simulink model "Golden_Model"  (R2025b)
settings: Solver=VariableStepAuto  StartTime=0.0  StopTime=20  RelTol=1e-3
undefined symbols (not defined in the file): b_mech, g, K_force, Kd_x_dummy, Ki_i_dummy, Kp_i_dummy, Kp_x_dummy, L, m, R_coil, R_eff
settings Model: Creator=nektariakaragiannis  LastModifiedBy=lucianbracy

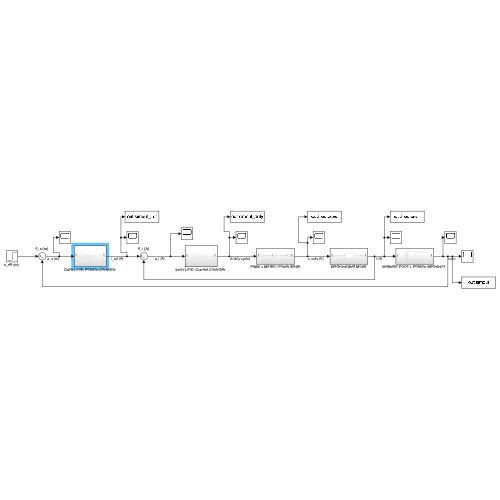
[thumbnail: Simulink's stored preview of the top-level diagram]
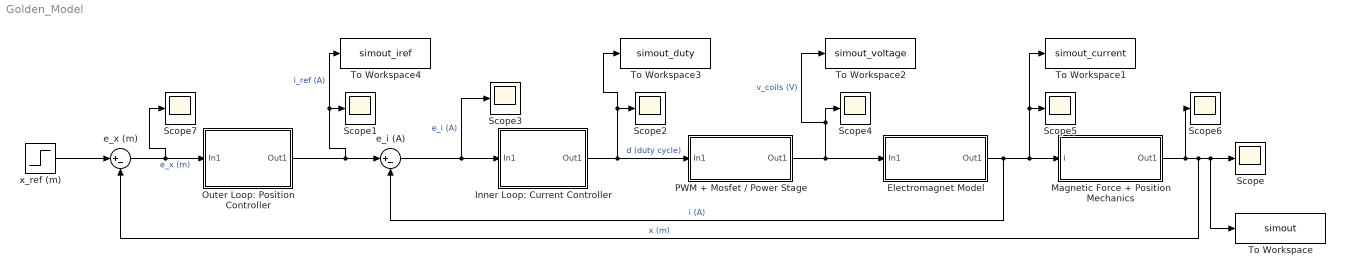
== system Golden_Model ==
  Electromagnet Model : Subsystem
  "Inner Loop: Current Controller " : Subsystem
  "Magnetic Force + Position Mechanics " : Subsystem
  Outer Loop: Position Controller : Subsystem
  PWM + Mosfet / Power Stage : Subsystem
  Scope{,1..7} (8 alike) : Scope
      Scope settings: ActiveDisplayYMinimum=-1  ActiveDisplayYMaximum=1
      Scope1 settings: ActiveDisplayYMinimum=-1  ActiveDisplayYMaximum=1  DataLoggingVariableName=ScopeData3
      Scope2 settings: ActiveDisplayYMinimum=-1  ActiveDisplayYMaximum=1  DataLoggingVariableName=ScopeData4
      Scope3 settings: ActiveDisplayYMinimum=-1  ActiveDisplayYMaximum=1  DataLoggingVariableName=ScopeData5
      Scope4 settings: ActiveDisplayYMinimum=-1  ActiveDisplayYMaximum=1  DataLoggingVariableName=ScopeData6
      Scope5 settings: ActiveDisplayYMinimum=-1  ActiveDisplayYMaximum=1  DataLoggingVariableName=ScopeData7
      Scope6 settings: ActiveDisplayYMinimum=-1  ActiveDisplayYMaximum=1  DataLoggingVariableName=ScopeData8
      Scope7 settings: ActiveDisplayYMinimum=-1  ActiveDisplayYMaximum=1  DataLoggingVariableName=ScopeData9
  To Workspace : ToWorkspace  VariableName=simout  SaveFormat=Timeseries  SampleTime=-1
  To Workspace1 : ToWorkspace  VariableName=simout_current  SaveFormat=Timeseries  SampleTime=-1
  To Workspace2 : ToWorkspace  VariableName=simout_voltage  SaveFormat=Timeseries  SampleTime=-1
  To Workspace3 : ToWorkspace  VariableName=simout_duty  SaveFormat=Timeseries  SampleTime=-1
  To Workspace4 : ToWorkspace  VariableName=simout_iref  SaveFormat=Timeseries  SampleTime=-1
  e_i (A) : Sum  Inputs=|+-
  e_x (m) : Sum  Inputs=|+-
  "x_ref (m) " : Step  After=0.0127  SampleTime=0
  wires:
  "x_ref (m) "/1 -> e_x (m)/1
  e_x (m)/1 -> Scope7/1, Outer Loop: Position Controller/1(In1)  "e_x (m)"
  Outer Loop: Position Controller/1(Out1) -> To Workspace4/1, Scope1/1, e_i (A)/1  "i_ref (A)"
  e_i (A)/1 -> Scope3/1, "Inner Loop: Current Controller "/1(In1)  "e_i (A)"
  "Inner Loop: Current Controller "/1(Out1) -> To Workspace3/1, Scope2/1, PWM + Mosfet / Power Stage/1(In1)  "d (duty cycle)"
  PWM + Mosfet / Power Stage/1(Out1) -> Scope4/1, To Workspace2/1, Electromagnet Model/1(In1)  "v_coils (V)"
  Electromagnet Model/1(Out1) -> e_i (A)/2, To Workspace1/1, Scope5/1, "Magnetic Force + Position Mechanics "/1(i)  "i (A)"
  "Magnetic Force + Position Mechanics "/1(Out1) -> Scope6/1, To Workspace/1, Scope/1, e_x (m)/2  "x (m)"

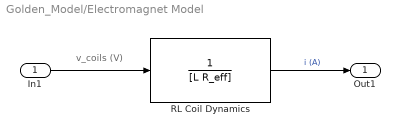
== system Golden_Model/Electromagnet Model ==
  note: v_coils (V)
  In1 : Inport
  RL Coil Dynamics : TransferFcn  Denominator=[L R_eff]
  Out1 : Outport
  wires:
  In1/1 -> RL Coil Dynamics/1
  RL Coil Dynamics/1 -> Out1/1  "i (A)"

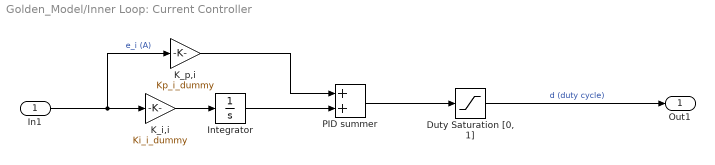
== system Golden_Model/Inner Loop: Current Controller  ==
  In1 : Inport
  "Duty Saturation [0, 1]" : Saturate  UpperLimit=1  LowerLimit=0
  Integrator : Integrator
  K_i,i : Gain  Gain=Ki_i_dummy
  K_p,i : Gain  Gain=Kp_i_dummy
  PID summer : Sum
  Out1 : Outport
  wires:
  K_p,i/1 -> PID summer/1
  Integrator/1 -> PID summer/2
  "Duty Saturation [0, 1]"/1 -> Out1/1  "d (duty cycle)"
  K_i,i/1 -> Integrator/1
  In1/1 -> K_p,i/1, K_i,i/1  "e_i (A)"
  PID summer/1 -> "Duty Saturation [0, 1]"/1

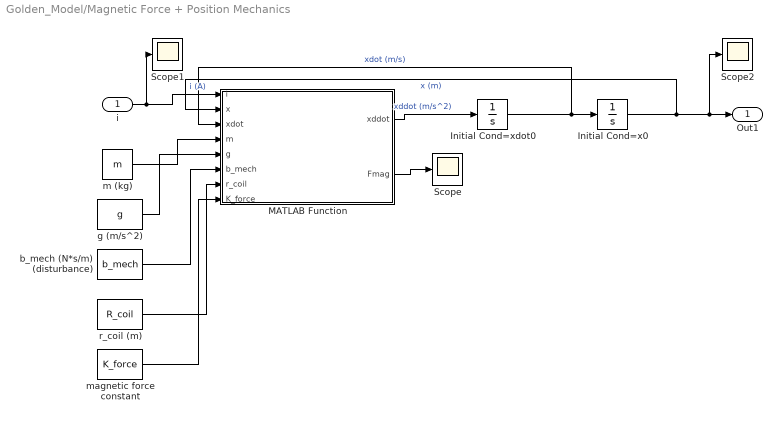
== system Golden_Model/Magnetic Force + Position Mechanics  ==
  i : Inport
  Initial Cond=x0 : Integrator  InitialCondition=0.0254  LimitOutput=on  UpperSaturationLimit=0.0254  LowerSaturationLimit=0
  Initial Cond=xdot0 : Integrator
  MATLAB Function : MATLAB Function  TreatAsAtomicUnit=on
  Scope : Scope
      settings: ActiveDisplayYMinimum=-10.345488701219102  ActiveDisplayYMaximum=93.109398310971926
  Scope1 : Scope
      settings: ActiveDisplayYMinimum=-1  ActiveDisplayYMaximum=1  DataLoggingVariableName=ScopeData2
  Scope2 : Scope
      settings: ActiveDisplayYMinimum=-2.3103125504803335  ActiveDisplayYMaximum=20.69509937729002  DataLoggingVariableName=ScopeData10
  b_mech (N*s/m) (disturbance) : Constant  Value=b_mech
  g (m/s^2) : Constant  Value=g
  m (kg) : Constant  Value=m
  magnetic force constant : Constant  Value=K_force
  r_coil (m) : Constant  Value=R_coil
  Out1 : Outport
  wires:
  i/1 -> Scope1/1, MATLAB Function/1(i)  "i (A)"
  MATLAB Function/1(xddot) -> Initial Cond=xdot0/1  "xddot (m/s^2)"
  Initial Cond=xdot0/1 -> MATLAB Function/3(xdot), Initial Cond=x0/1  "xdot (m/s)"
  Initial Cond=x0/1 -> MATLAB Function/2(x), Scope2/1, Out1/1  "x (m)"
  MATLAB Function/2(Fmag) -> Scope/1
  m (kg)/1 -> MATLAB Function/4(m)
  g (m/s^2)/1 -> MATLAB Function/5(g)
  b_mech (N*s/m) (disturbance)/1 -> MATLAB Function/6(b_mech)
  r_coil (m)/1 -> MATLAB Function/7(r_coil)
  magnetic force constant/1 -> MATLAB Function/8(K_force)

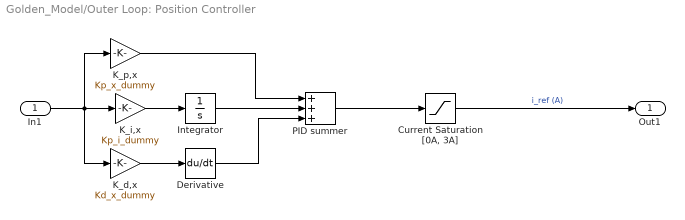
== system Golden_Model/Outer Loop: Position Controller ==
  In1 : Inport
  "Current Saturation [0A, 3A]" : Saturate  UpperLimit=5  LowerLimit=0
  Derivative : Derivative
  Integrator : Integrator  InitialCondition=0.0254
  K_d,x : Gain  Gain=Kd_x_dummy
  K_i,x : Gain  Gain=Kp_i_dummy
  K_p,x : Gain  Gain=Kp_x_dummy
  PID summer : Sum  Inputs=+++
  Out1 : Outport
  wires:
  PID summer/1 -> "Current Saturation [0A, 3A]"/1
  In1/1 -> K_p,x/1, K_i,x/1, K_d,x/1
  K_i,x/1 -> Integrator/1
  K_d,x/1 -> Derivative/1
  Integrator/1 -> PID summer/2
  K_p,x/1 -> PID summer/1
  Derivative/1 -> PID summer/3
  "Current Saturation [0A, 3A]"/1 -> Out1/1  "i_ref (A)"

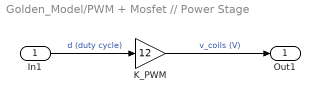
== system Golden_Model/PWM + Mosfet // Power Stage ==
  In1 : Inport
  K_PWM : Gain  Gain=12
  Out1 : Outport
  wires:
  In1/1 -> K_PWM/1  "d (duty cycle)"
  K_PWM/1 -> Out1/1  "v_coils (V)"

== matlab function Golden_Model/Magnetic Force + Position Mechanics /MATLAB Function ==
  data: i input; xddot output; x input; xdot input; Fmag output; m input; g input; b_mech input; r_coil input; K_force input
function [xddot, Fmag] = maglev_force(i, x, xdot, m, g, b_mech, r_coil, K_force)
%x_safe = max(x, r_coil/2); % cannot closer than half coil radius
x_safe = max(x, 1e-4);

Fmag = (K_force * i * x_safe) / ((x_safe^2 + r_coil^2)^(5/2));

xddot = g - Fmag/m - b_mech*xdot/m;
